simulink model "Copy_of_vehicle"  (R2021a)
settings: Solver=VariableStepAuto  StartTime=0  StopTime=80  RelTol=1e-3
values from neighbouring files (symbols this model uses):
  Ld = 0.3e-3    (= 0.0003)    [PMSM_paramaters.m]
  Lq = 0.4e-3    (= 0.0004)    [PMSM_paramaters.m]
  P = 4    [PMSM_paramaters.m]
  Pm = 0.15    [PMSM_paramaters.m]
  Rs = 0.03    [PMSM_paramaters.m]
  T_lookup = [289,289,0]    [PMSM_paramaters.m]
  Torque = 289    [PMSM_paramaters.m]
  Ts = 1e-2    (= 0.01)    [PMSM_paramaters.m]
undefined symbols (not defined in the file or in its folder): sigbuilder_block
libraries: pid_lib x3, simulink x3, autolibshared x1, simulink_extras x1, spspowerguiLib x1
settings Model: SimulationMode=accelerator  Creator=user  LastModifiedBy=USER
settings DebuggingCC: SFMachineParentedDataDiag=warning

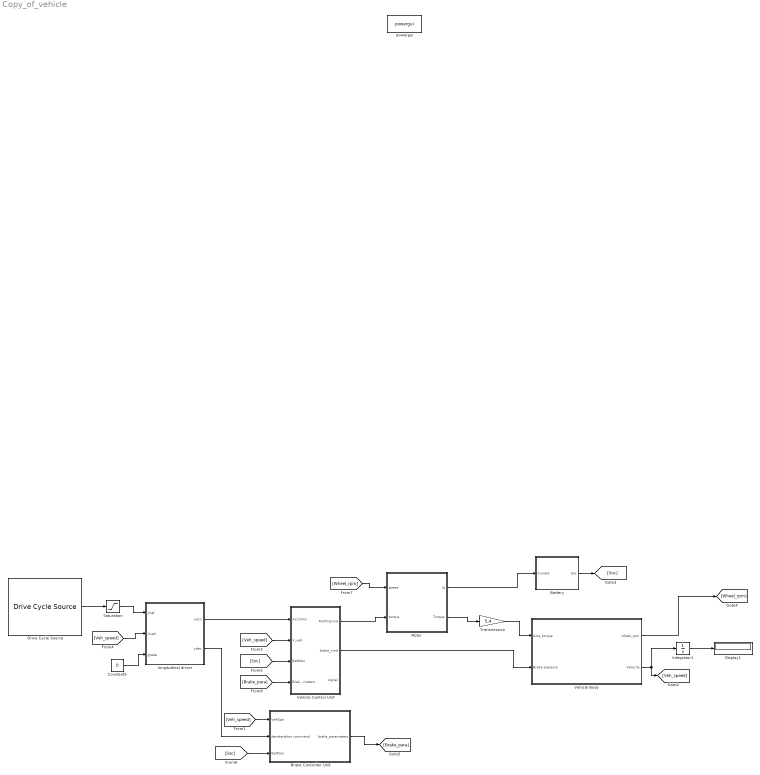
== system Copy_of_vehicle ==
  Battery : Subsystem
  Brake Controller Unit : Subsystem
  Constant5 : Constant  Value=0
  Display1 : Display
  Drive Cycle Source : autolibshared/Drive Cycle Source  cycleVar=Wide Open Throttle (WOT)  fileVar=cycleFTP75.mat  tfinal="300  seconds"  cycleRepeat=off  outAccPort=off  outGearPort=off  gearList=No gear data  t_wot1=0.1  xdot_woto=0  xdot_wot1=10.4  t_wot2=20  xdot_wot2=0  t_wotend=300  srcUnit=m/s  outUnit=m/s  srcAccUnit=m/s/s  outAccUnit=m/s^2  dt=0  aMode=1  faultOption=off  velBnd=2  velBndUnit=mph  inUnit=m/s  timeBnd=1  failOption=off  stopSim=off  maxFaultCnt=10  maxFaultTime=2  maxTotFaultTime=15  traceOption=off  dtTrace=1  traceWindow=10  lastDCname=Custom Data Set  lastOutUnit=mph  lastDT=0  lastTB=1  lastSB=2  forceCalcBound=off
      settings: SourceProductBaseCode=PW,DR,MT,UV,VE
  Integrator1 : Integrator
  Motor : Subsystem
  Saturation : Saturate  UpperLimit=50  LowerLimit=0
  Transmission : Gain  Gain=5.4
      settings: AttributesFormatString=%<Gain>
  Vehicle Body : Subsystem
  Vehicle Control Unit : Subsystem
  longitudinal driver : Subsystem
  powergui : spspowerguiLib/powergui  Priority=1  SimulationMode=Continuous  SampleTime=50e-6  frequency=60  Iterations=50  frequencyindice=0  Pbase=100e6  ErrMax=1e-4  UnitsV=kV  UnitsW=MW  buscounter=0  FunctionMessages=off  echomessages=off  EnableUseOfTLC=off  CurrentSourceSwitches=off  DisableSnubberDevices=off  DisableRonSwitches=off  DisableVfSwitches=off  DisplayEquations=off  AutomaticDiscreteSolvers=off  SolverType=Tustin/Backward Euler (TBE)  Interpol=off  ExternalGateDelay=off  methode=off  Ts=100  x0status=blocks  SPID=on  SwTol=0  HookPort=off  NonlinearTolerance=1e-4  nMaxIteration=100  ContinueOnMaxIteration=off  RestoreLinks=warning  ResistiveCurrentMeasurement=off  Frange=[0:2:500]  Ylog=off  Xlog=on  ShowGrid=off  save=off  variable=ZData  structure=0  ZoomFFT=off  StartTime=0.0  cycles=1  DisplayStyle=1  fundamental=60  FreqAxis=off  MaxFrequency=1000  frequencyindicesteady=1  RmsSteady=1  display=off
  wires:
  Drive Cycle Source/1 -> Saturation/1
  Integrator1/1 -> Display1/1
  Constant5/1 -> longitudinal driver/3(grade)
  Saturation/1 -> longitudinal driver/1(Vref)
  longitudinal driver/1(yacc) -> Vehicle Control Unit/1(AccCmd)
  longitudinal driver/2(ydec) -> Brake Controller Unit/2("deceleration command ")
  Vehicle Control Unit/2(brake_cmd) -> Vehicle Body/2(Brake pressure)
  Vehicle Body/2(Velocity) -> Integrator1/1, [Veh_speed]
  Transmission/1 -> Vehicle Body/1(Axle_torque)
  Vehicle Body/1(wheel_rpm) -> [Wheel_rpm]
  Brake Controller Unit/1(" brake_parameters") -> [Brake_para]
  Battery/1(Soc) -> [Soc]
  [Veh_speed] -> Brake Controller Unit/1(VehSpd)
  [Veh_speed] -> longitudinal driver/2(Vveh)
  [Veh_speed] -> Vehicle Control Unit/2(V_veh)
  [Soc] -> Vehicle Control Unit/3(BattSoc)
  [Soc] -> Brake Controller Unit/3(BattSoc)
  [Wheel_rpm] -> Motor/1(speed)
  Vehicle Control Unit/1(MotTrqCmd) -> Motor/2(torque)
  Motor/2(Torque) -> Transmission/1
  [Brake_para] -> Vehicle Control Unit/4(Brake_parameters)
  Motor/1(Iq) -> Battery/1(Current)

== system Copy_of_vehicle/Battery ==
  Current : Inport
  Constant : Constant
  Convert to Ah : Gain  Gain=-1/3600
  Convert to SOC : Gain  Gain=1/30200
  Integrator : Integrator
  e-ref : Sum
  Soc : Outport
  wires:
  Integrator/1 -> Convert to SOC/1
  Convert to Ah/1 -> Integrator/1
  Current/1 -> Convert to Ah/1
  Constant/1 -> e-ref/1
  Convert to SOC/1 -> e-ref/2
  e-ref/1 -> Soc/1

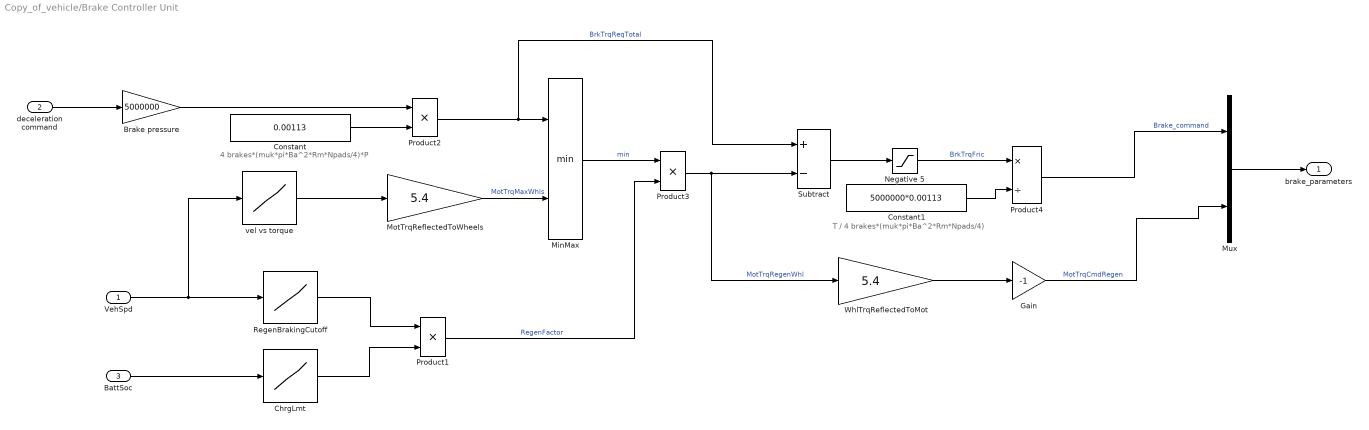
== system Copy_of_vehicle/Brake Controller Unit ==
  note: T / 4 brakes*(muk*pi*Ba^2*Rm*Npads/4)
  note: 4 brakes*(muk*pi*Ba^2*Rm*Npads/4)*P
  VehSpd : Inport
  "deceleration command " : Inport  Port=2
  BattSoc : Inport  Port=3
  Brake pressure : Gain  Gain=5000000
  ChrgLmt : Lookup_n-D  NumberOfTableDimensions=1  BreakpointsForDimension1=[0 10 20 30 40 50 60 70 80 90 100]  Table=[1 1 1 1 1 1 1 1 0.7 0.35 0]  ExtrapMethod=Clip  UseLastTableValue=on  InternalRulePriority=Speed  RndMeth=Simplest  InputSameDT=on
  Constant : Constant  Value=0.00113
  Constant1 : Constant  Value=5000000*0.00113
  Gain : Gain  Gain=-1
  MinMax : MinMax  Inputs=2
  MotTrqReflectedToWheels : Gain  Gain=5.4
  Mux : Mux  Inputs=2
  Negative 5 : Saturate  UpperLimit=inf  LowerLimit=0
  Product1 : Product
  Product2 : Product
  Product3 : Product
  Product4 : Product  Inputs=*/
  RegenBrakingCutoff : Lookup_n-D  NumberOfTableDimensions=1  BreakpointsForDimension1=[5 9]  Table=[0 1]  ExtrapMethod=Clip  UseLastTableValue=on  InternalRulePriority=Speed  RndMeth=Simplest  InputSameDT=on
  Subtract : Sum  Inputs=+-
  WhlTrqReflectedToMot : Gain  Gain=5.4
  vel vs torque : Lookup_n-D  NumberOfTableDimensions=1  BreakpointsForDimension1=[0 , 27.78,150]  Table=[286,286,0]  InternalRulePriority=Speed  RndMeth=Simplest  InputSameDT=on
  " brake_parameters" : Outport  VectorParamsAs1DForOutWhenUnconnected=off
  wires:
  Subtract/1 -> Negative 5/1
  Constant1/1 -> Product4/2
  MinMax/1 -> Product3/1  "min"
  BattSoc/1 -> ChrgLmt/1
  VehSpd/1 -> vel vs torque/1, RegenBrakingCutoff/1
  MotTrqReflectedToWheels/1 -> MinMax/2  "MotTrqMaxWhls"
  Constant/1 -> Product2/2
  "deceleration command "/1 -> Brake pressure/1
  Product2/1 -> MinMax/1, Subtract/1  "BrkTrqReqTotal"
  ChrgLmt/1 -> Product1/2
  RegenBrakingCutoff/1 -> Product1/1
  Product1/1 -> Product3/2  "RegenFactor"
  Negative 5/1 -> Product4/1  "BrkTrqFric"
  Mux/1 -> " brake_parameters"/1
  Product3/1 -> WhlTrqReflectedToMot/1, Subtract/2  "MotTrqRegenWhl"
  Gain/1 -> Mux/2  "MotTrqCmdRegen"
  WhlTrqReflectedToMot/1 -> Gain/1
  Product4/1 -> Mux/1  "Brake_command"
  Brake pressure/1 -> Product2/1
  vel vs torque/1 -> MotTrqReflectedToWheels/1

== system Copy_of_vehicle/Motor ==
  speed : Inport
  torque : Inport  Port=2
  1 : Gain  Gain=5.4
      settings: AttributesFormatString=%<Gain>
  FOC : Subsystem
  PMSM : Subsystem
  Unit Delay : UnitDelay  SampleTime=Ts  HasFrameUpgradeWarning=on
  Iq : Outport
  Torque : Outport  Port=2
  wires:
  torque/1 -> FOC/3(torque)
  FOC/1(Vabc) -> PMSM/1(Vabc)
  speed/1 -> 1/1
  PMSM/1(Iabc) -> FOC/2(Iabc)
  PMSM/3(Iq) -> Iq/1  "Iq"
  PMSM/2(Torque) -> Torque/1
  Unit Delay/1 -> FOC/4(Vdq)
  PMSM/4(Vdq) -> Unit Delay/1
  1/1 -> [Motor_speed]
  [Motor_speed] -> FOC/1(RotorSpeed_fbk)
  [Motor_speed] -> PMSM/2(speed)

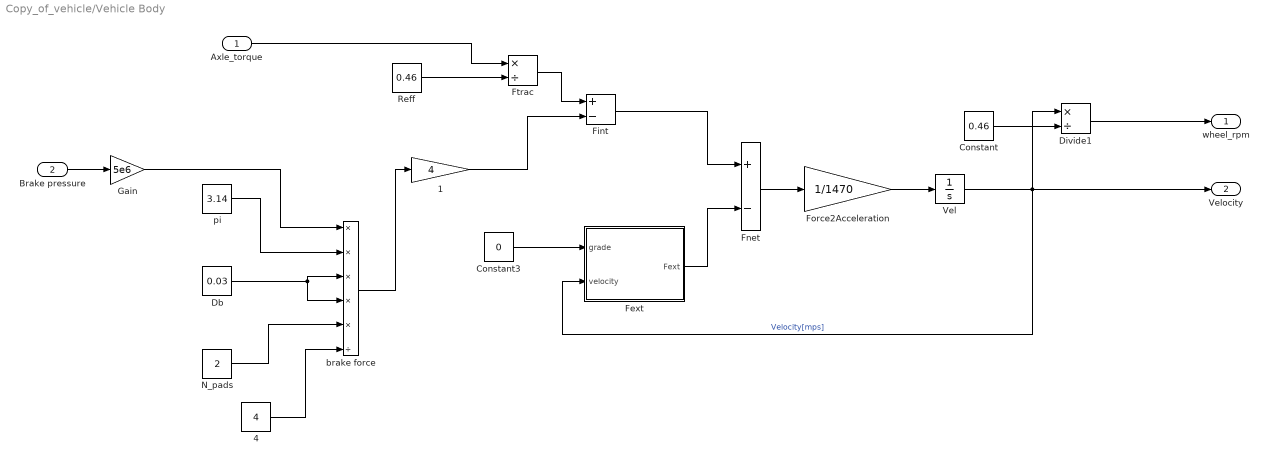
== system Copy_of_vehicle/Vehicle Body ==
  Axle_torque : Inport
  Brake pressure : Inport  Port=2
  1 : Gain  Gain=4
      settings: AttributesFormatString=%<Gain>
  4 : Constant  Value=4
  Constant : Constant  Value=0.46
  Constant3 : Constant  Value=0
  Db : Constant  Value=0.03
  Divide1 : Product  Inputs=*/
  Fext : Subsystem
  Fint : Sum  Inputs=+-
  Fnet : Sum  Inputs=+-
  Force2Acceleration : Gain  Gain=1/1470
      settings: AttributesFormatString=%<Gain>
  Ftrac : Product  Inputs=*/
  Gain : Gain  Gain=5e6
  N_pads : Constant  Value=2
  Reff : Constant  Value=0.46
  Vel : Integrator
  brake force : Product  Inputs=*****/
  pi : Constant  Value=3.14
  wheel_rpm : Outport
  Velocity : Outport  Port=2
  wires:
  Ftrac/1 -> Fint/1
  Fnet/1 -> Force2Acceleration/1
  Fext/1(Fext) -> Fnet/2
  Vel/1 -> Velocity/1, Divide1/1, Fext/2(velocity)  "Velocity[mps]"
  Reff/1 -> Ftrac/2
  Constant3/1 -> Fext/1(grade)
  Brake pressure/1 -> Gain/1
  Fint/1 -> Fnet/1
  Axle_torque/1 -> Ftrac/1
  1/1 -> Fint/2
  Force2Acceleration/1 -> Vel/1
  Constant/1 -> Divide1/2
  Divide1/1 -> wheel_rpm/1
  brake force/1 -> 1/1
  Gain/1 -> brake force/1
  4/1 -> brake force/6
  Db/1 -> brake force/3, brake force/4
  pi/1 -> brake force/2
  N_pads/1 -> brake force/5

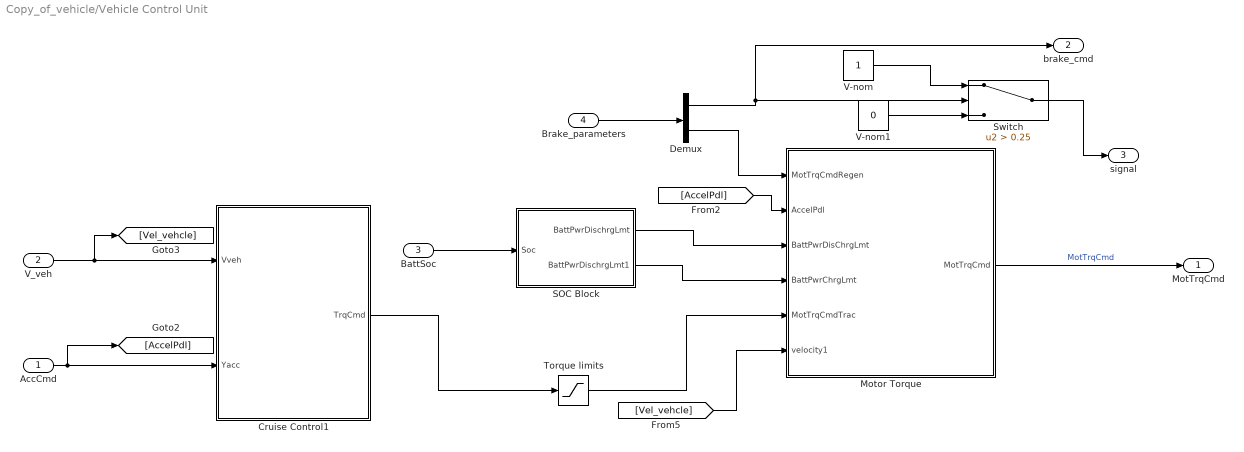
== system Copy_of_vehicle/Vehicle Control Unit ==
  AccCmd : Inport
  V_veh : Inport  Port=2
  BattSoc : Inport  Port=3
  Brake_parameters : Inport  Port=4
  Cruise Control1 : Subsystem
  Demux : Demux  Outputs=2
  "Motor Torque " : Subsystem
  SOC Block : Subsystem
  Switch : Switch  Criteria=u2 > Threshold  Threshold=0.25
  Torque limits : Saturate  UpperLimit=Torque  LowerLimit=0
  V-nom : Constant
  V-nom1 : Constant  Value=0
  MotTrqCmd : Outport
  brake_cmd : Outport  Port=2
  signal : Outport  Port=3
  wires:
  Torque limits/1 -> "Motor Torque "/5(MotTrqCmdTrac)
  V_veh/1 -> Cruise Control1/1(Vveh), [Vel_vehcle]
  Cruise Control1/1(TrqCmd) -> Torque limits/1
  AccCmd/1 -> Cruise Control1/2(Yacc), [AccelPdl]
  SOC Block/1(BattPwrDischrgLmt) -> "Motor Torque "/3(BattPwrDisChrgLmt)
  BattSoc/1 -> SOC Block/1(Soc)
  SOC Block/2(BattPwrDischrgLmt1) -> "Motor Torque "/4("BattPwrChrgLmt ")
  "Motor Torque "/1(MotTrqCmd) -> MotTrqCmd/1  "MotTrqCmd"
  [Vel_vehcle] -> "Motor Torque "/6(velocity1)
  [AccelPdl] -> "Motor Torque "/2(AccelPdl)
  Brake_parameters/1 -> Demux/1
  Demux/2 -> "Motor Torque "/1(MotTrqCmdRegen)
  Demux/1 -> brake_cmd/1, Switch/2
  V-nom1/1 -> Switch/3
  V-nom/1 -> Switch/1
  Switch/1 -> signal/1

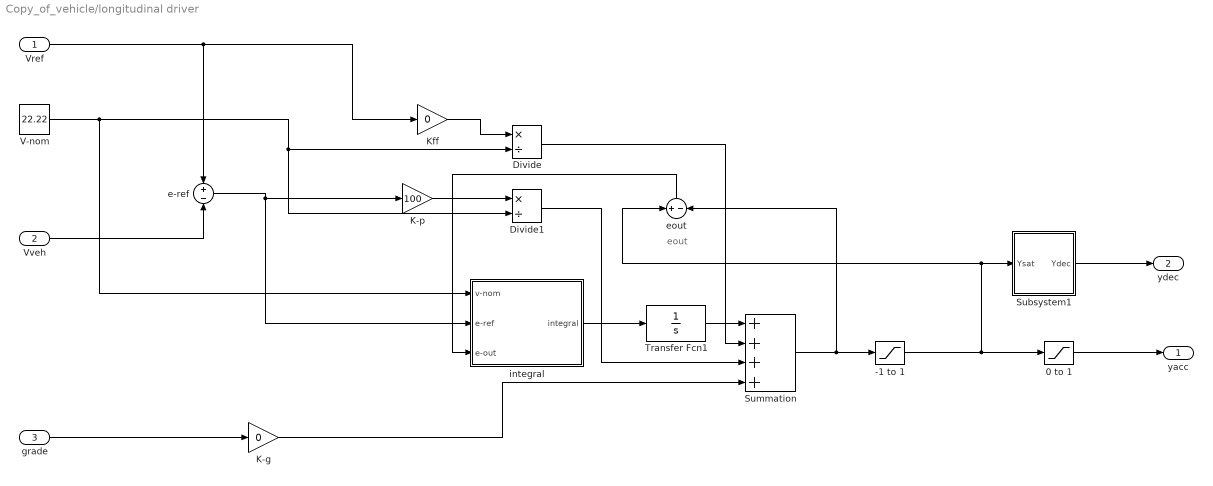
== system Copy_of_vehicle/longitudinal driver ==
  note: eout
  Vref : Inport
  Vveh : Inport  Port=2
  grade : Inport  Port=3
  "-1 to 1 " : Saturate  UpperLimit=1  LowerLimit=-1
  0 to 1 : Saturate  UpperLimit=1  LowerLimit=0
  Divide : Product  Inputs=*/
  Divide1 : Product  Inputs=*/
  K-g : Gain  Gain=0
  K-p : Gain  Gain=100
  Kff : Gain  Gain=0
  Subsystem1 : Subsystem
  Summation : Sum  Inputs=++++
  Transfer Fcn1 : TransferFcn  Denominator=[1 0]
  V-nom : Constant  Value=22.22
  e-ref : Sum  Inputs=+-
  eout : Sum  Inputs=+-
  integral : Subsystem
  yacc : Outport
  ydec : Outport  Port=2
  wires:
  V-nom/1 -> Divide1/2, Divide/2, integral/1(v-nom)
  e-ref/1 -> K-p/1, integral/2(e-ref)
  Divide/1 -> Summation/2
  Summation/1 -> "-1 to 1 "/1, eout/2
  Vref/1 -> Kff/1, e-ref/1
  integral/1(integral) -> Transfer Fcn1/1
  K-p/1 -> Divide1/1
  Transfer Fcn1/1 -> Summation/1
  Kff/1 -> Divide/1
  eout/1 -> integral/3(e-out)
  Vveh/1 -> e-ref/2
  Divide1/1 -> Summation/3
  grade/1 -> K-g/1
  Subsystem1/1(Ydec) -> ydec/1
  0 to 1/1 -> yacc/1
  K-g/1 -> Summation/4
  "-1 to 1 "/1 -> 0 to 1/1, Subsystem1/1(Ysat), eout/1

== system Copy_of_vehicle/Motor/FOC ==
  RotorSpeed_fbk : Inport
  Iabc : Inport  Port=2
  torque : Inport  Port=3
  Vdq : Inport  Port=4
  Inverse - Park1 : Subsystem
  Inverse Clarke1 : Subsystem
  Subsystem2 : Subsystem
  clarke : Subsystem
  current controller : Subsystem
  park : Subsystem
  torque_Idq_ref : Subsystem
  Vabc : Outport
  wires:
  [theta] -> Inverse - Park1/2(theta)
  RotorSpeed_fbk/1 -> [Omega], Subsystem2/1(omega)
  Inverse - Park1/2(V-beta) -> Inverse Clarke1/2(Vbeta)
  Iabc/1 -> clarke/1(Iabc)
  torque/1 -> torque_Idq_ref/1(Torque)
  Inverse - Park1/1(V-alpha) -> Inverse Clarke1/1(Valpha)
  current controller/2(Vq) -> Inverse - Park1/3(Vq)
  park/1(Id) -> current controller/2(Id), torque_Idq_ref/2(Id)
  current controller/1(Vd) -> Inverse - Park1/1(Vd)
  Subsystem2/1(theta_deg) -> park/2(theta), [theta]
  torque_Idq_ref/1(Id_ref) -> current controller/1(Id_ref)
  park/2(Iq) -> current controller/4(Iq)
  [Omega] -> current controller/3(omega)
  torque_Idq_ref/2(Iq_ref) -> current controller/5(Iq_ref)
  clarke/1(I_alpha) -> park/1(I_alpha)
  Inverse Clarke1/1(Vabc) -> Vabc/1
  clarke/2(I_beta) -> park/3(I_beta)
  Vdq/1 -> torque_Idq_ref/3(Vdq)

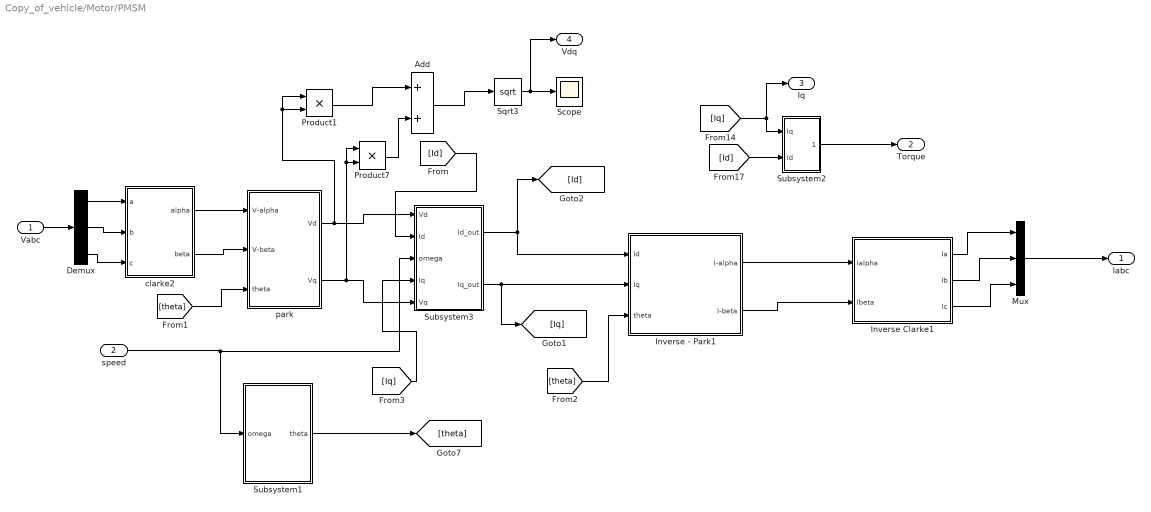
== system Copy_of_vehicle/Motor/PMSM ==
  Vabc : Inport
  speed : Inport  Port=2
  Add : Sum
  Demux : Demux  Outputs=3
  Inverse - Park1 : Subsystem
  Inverse Clarke1 : Subsystem
  Mux : Mux  Inputs=3
  Product1 : Product
  Product7 : Product
  Scope : Scope
  Sqrt3 : Sqrt  SaturateOnIntegerOverflow=on
  Subsystem1 : Subsystem
  Subsystem2 : Subsystem
  Subsystem3 : Subsystem
  clarke2 : Subsystem
  park : Subsystem
  Iabc : Outport
  Torque : Outport  Port=2
  Iq : Outport  Port=3
  Vdq : Outport  Port=4
  wires:
  Mux/1 -> Iabc/1
  Demux/1 -> clarke2/1(a)
  Vabc/1 -> Demux/1
  Inverse - Park1/2(I-beta) -> Inverse Clarke1/2(Ibeta)
  Subsystem3/1(Id_out) -> Inverse - Park1/1(Id), [Id]
  Inverse Clarke1/1(Ia) -> Mux/1
  Demux/3 -> clarke2/3(c)
  Demux/2 -> clarke2/2(b)
  Subsystem1/1(theta) -> [theta]
  Inverse Clarke1/2(Ib) -> Mux/2
  clarke2/2(beta) -> park/2(V-beta)
  [Id] -> Subsystem3/2(Id)
  Subsystem3/2(Iq_out) -> Inverse - Park1/2(Iq), [Iq]
  clarke2/1(alpha) -> park/1(V-alpha)
  park/2(Vq) -> Subsystem3/5(Vq), Product7/1, Product7/2
  Inverse Clarke1/3(Ic) -> Mux/3
  Inverse - Park1/1(I-alpha) -> Inverse Clarke1/1(Ialpha)
  park/1(Vd) -> Product1/2, Product1/1, Subsystem3/1(Vd)
  [Id] -> Subsystem2/2(Id)
  [theta] -> park/3(theta)
  [Iq] -> Iq/1, Subsystem2/1(Iq)
  Subsystem2/1(Torque) -> Torque/1
  [theta] -> Inverse - Park1/3(theta)
  speed/1 -> Subsystem1/1(omega), Subsystem3/3(omega)
  [Iq] -> Subsystem3/4(Iq)
  Product7/1 -> Add/2
  Product1/1 -> Add/1
  Add/1 -> Sqrt3/1
  Sqrt3/1 -> Vdq/1, Scope/1

== system Copy_of_vehicle/Vehicle Body/Fext ==
  grade : Inport
  velocity : Inport  Port=2
  Cd1 : Constant  Value=0.38  OutDataTypeStr=single
  Cd2 : Constant  Value=2.27  OutDataTypeStr=single
  Cos : Trigonometry  Operator=cos
  Sum : Sum  Inputs=+++
  Trigonometric Function : Trigonometry
  aero : Product  Inputs=6
  coeff_fric : Constant  Value=0.01  OutDataTypeStr=single
  constant : Constant  Value=0.5  OutDataTypeStr=single
  density : Constant  Value=1.2  OutDataTypeStr=single
  g : Constant  Value=9.81  OutDataTypeStr=single
  g1 : Constant  OutDataTypeStr=single
  g2 : Constant  Value=9.81  OutDataTypeStr=single
  gradient_force : Product  Inputs=3
  mass : Constant  Value=1470  OutDataTypeStr=single
  rolling_res : Product  Inputs=5
  Fext : Outport
  wires:
  g2/1 -> gradient_force/2
  mass/1 -> gradient_force/3, rolling_res/1
  Trigonometric Function/1 -> gradient_force/1
  g/1 -> rolling_res/2
  g1/1 -> rolling_res/3
  grade/1 -> Cos/1, Trigonometric Function/1
  coeff_fric/1 -> rolling_res/4
  Cd1/1 -> aero/4
  density/1 -> aero/2
  constant/1 -> aero/1
  Cd2/1 -> aero/5
  velocity/1 -> aero/3, aero/6
  gradient_force/1 -> Sum/1
  aero/1 -> Sum/2
  rolling_res/1 -> Sum/3
  Sum/1 -> Fext/1
  Cos/1 -> rolling_res/5

== system Copy_of_vehicle/Vehicle Control Unit/Cruise Control1 ==
  Vveh : Inport
  Yacc : Inport  Port=2
  Capture speed : Subsystem  TreatAsAtomicUnit=on
  Constant5 : Constant  Value=0
  Data Type Conversion1 : DataTypeConversion  OutDataTypeStr=boolean
  Data Type Conversion2 : DataTypeConversion  OutDataTypeStr=boolean
  Data Type Conversion3 : DataTypeConversion  OutDataTypeStr=boolean
  Inputs1 : Subsystem  Tag=STV Subsys  LoadFcn=sigbuilder_block('load');  StartFcn=sigbuilder_block('start');  StopFcn=sigbuilder_block('stop');  ClipboardFcn=sigbuilder_block('clipboard');  mask(Sigbuilder block){tuvar=[0:10]}
      mask help: Simulink:masks:SigbuilderBlock_MD
      mask init:
      | if ~strcmp(get_param(bdroot(gcbh),'SimulationStatus'),'stopped') tuvar = sigbuilder_block('maskInit'); end
      settings: CopyFcn=sigbuilder_block('copy');  DeleteFcn=sigbuilder_block('delete');  ModelCloseFcn=sigbuilder_block('modelClose');  PreSaveFcn=sigbuilder_block('preSave');  PauseFcn=sigbuilder_block('pause');  ContinueFcn=sigbuilder_block('continue');  NameChangeFcn=sigbuilder_block('namechange');  OpenFcn=sigbuilder_block('open',[5.4 30 1141.2 522.6 ]);  CloseFcn=sigbuilder_block('close');
      mask Display: plot(0, 0, 100, 100,[2, 2, 32, 32, 2], [68, 8, 8, 68, 68],[32, 2], [38, 38], [32, 19, 2],[53, 60, 44], [32, 17, 17, 2],[16, 16, 31, 31]);txt = getActiveGroup(gcbh);text(2, 100, txt,'verticalAlignment', 'top');
  J-K Flip-Flop : simulink_extras/Flip Flops/J-K Flip-Flop  initial_condition=0
      settings: SourceProductName=Simulink Extras
  Pulse Generator : DiscretePulseGenerator  Period=10  PulseWidth=5  SampleTime=0.01
  Subsystem : Subsystem
  Switch : Switch  Criteria=u2 > Threshold
  Terminator : Terminator
  longitudinal driver : Subsystem
  TrqCmd : Outport  VectorParamsAs1DForOutWhenUnconnected=off
  wires:
  Inputs1/1(Cruise Ena.) -> Data Type Conversion1/1
  Pulse Generator/1 -> Data Type Conversion2/1
  J-K Flip-Flop/1 -> Switch/2, Capture speed/Trigger
  Data Type Conversion1/1 -> J-K Flip-Flop/1
  J-K Flip-Flop/2 -> Terminator/1
  Capture speed/1(Vref) -> longitudinal driver/1(Vref)
  Inputs1/2(Cruise Dis.) -> Data Type Conversion3/1
  Yacc/1 -> Switch/3
  longitudinal driver/1(yacc) -> Switch/1
  Constant5/1 -> longitudinal driver/3(grade)
  Switch/1 -> Subsystem/1(Acc_pedal)
  Vveh/1 -> Capture speed/1(Vveh), Subsystem/2(velocity), longitudinal driver/2(Vveh)
  Subsystem/1(Torque_cmd) -> TrqCmd/1
  Data Type Conversion2/1 -> J-K Flip-Flop/2
  Data Type Conversion3/1 -> J-K Flip-Flop/3

== system Copy_of_vehicle/Vehicle Control Unit/Motor Torque  ==
  MotTrqCmdRegen : Inport
  AccelPdl : Inport  Port=2
  BattPwrDisChrgLmt : Inport  Port=3
  "BattPwrChrgLmt " : Inport  Port=4
  MotTrqCmdTrac : Inport  Port=5
  velocity1 : Inport  Port=6
  Accel Decel Switch : Switch  Criteria=u2 > Threshold
  Compare To Constant : simulink/Logic and Bit Operations/Compare To Constant  relop=>  const=0  OutDataTypeStr=boolean
  Gain : Gain  Gain=-1
  Saturation Dynamic : simulink/Discontinuities/Saturation Dynamic  OutMin=[]  OutMax=[]  OutDataTypeStr=Inherit: Same as second input  OutDataType=fixdt(1, 16)  OutScaling=2^-10  DoSatur=off
  Saturation Dynamic1 : simulink/Discontinuities/Saturation Dynamic  OutMin=[]  OutMax=[]  OutDataTypeStr=Inherit: Same as second input  OutDataType=fixdt(1, 16)  OutScaling=2^-10  DoSatur=off
  Vel vs Torque : Lookup_n-D  NumberOfTableDimensions=1  BreakpointsForDimension1=[0 , 27.78,50]  Table=T_lookup  InternalRulePriority=Speed  RndMeth=Simplest  InputSameDT=on
  MotTrqCmd : Outport
  wires:
  AccelPdl/1 -> Compare To Constant/1
  MotTrqCmdRegen/1 -> Accel Decel Switch/3
  MotTrqCmdTrac/1 -> Accel Decel Switch/1
  Accel Decel Switch/1 -> Saturation Dynamic1/2
  Compare To Constant/1 -> Accel Decel Switch/2
  Gain/1 -> Saturation Dynamic/3
  "BattPwrChrgLmt "/1 -> Saturation Dynamic1/3
  BattPwrDisChrgLmt/1 -> Saturation Dynamic1/1
  Saturation Dynamic1/1 -> Saturation Dynamic/2
  velocity1/1 -> Vel vs Torque/1
  Saturation Dynamic/1 -> MotTrqCmd/1
  Vel vs Torque/1 -> Saturation Dynamic/1, Gain/1

== system Copy_of_vehicle/Vehicle Control Unit/SOC Block ==
  Soc : Inport
  ChrgLmt : Lookup_n-D  NumberOfTableDimensions=1  BreakpointsForDimension1=[0 10 20 30 40 50 60 70 80 90 100]  Table=[1 1 1 1 1 1 1 1 0.7 0.35 0]  ExtrapMethod=Clip  UseLastTableValue=on  InternalRulePriority=Speed  RndMeth=Simplest  InputSameDT=on
  DischrgLmt : Lookup_n-D  NumberOfTableDimensions=1  BreakpointsForDimension1=[0 10 20 30 40 50 60 70 80 90 100]  Table=[0 0.35 0.7 1 1 1 1 1 1 1 1]  ExtrapMethod=Clip  UseLastTableValue=on  InternalRulePriority=Speed  RndMeth=Simplest  InputSameDT=on
  MaxChrg : Constant  Value=96234
  MaxChrg1 : Constant  Value=-96234
  Product : Product
  Product1 : Product
  BattPwrDischrgLmt : Outport  VectorParamsAs1DForOutWhenUnconnected=off
  BattPwrDischrgLmt1 : Outport  Port=2  VectorParamsAs1DForOutWhenUnconnected=off
  wires:
  Soc/1 -> DischrgLmt/1, ChrgLmt/1
  Product1/1 -> BattPwrDischrgLmt1/1
  Product/1 -> BattPwrDischrgLmt/1
  MaxChrg1/1 -> Product1/2
  ChrgLmt/1 -> Product1/1
  MaxChrg/1 -> Product/2
  DischrgLmt/1 -> Product/1

== system Copy_of_vehicle/longitudinal driver/Subsystem1 ==
  Ysat : Inport
  -2 : Constant  Value=0
  -5 : Constant
  K-p1 : Gain  Gain=-1
  K-p2 : Gain  Gain=-1
  Switch5 : Switch  Criteria=u2 > Threshold
  Switch6 : Switch  Threshold=-1
  Ydec : Outport
  wires:
  Switch5/1 -> Switch6/1, K-p2/1
  K-p1/1 -> Switch5/3
  Switch6/1 -> Ydec/1
  Ysat/1 -> Switch5/2, K-p1/1
  K-p2/1 -> Switch6/2
  -2/1 -> Switch5/1
  -5/1 -> Switch6/3

== system Copy_of_vehicle/longitudinal driver/integral ==
  v-nom : Inport
  e-ref : Inport  Port=2
  e-out : Inport  Port=3
  Divide2 : Product  Inputs=*/
  K-aw : Gain  Gain=0
  Ki : Gain
  Sum2 : Sum  Inputs=|++
  integral : Outport
  wires:
  Divide2/1 -> Sum2/1
  v-nom/1 -> Divide2/2
  e-ref/1 -> Ki/1
  K-aw/1 -> Sum2/2
  Ki/1 -> Divide2/1
  e-out/1 -> K-aw/1
  Sum2/1 -> integral/1

== system Copy_of_vehicle/Motor/FOC/Inverse - Park1 ==
  Vd : Inport
  theta : Inport  Port=2
  Vq : Inport  Port=3
  Cos : Trigonometry  Operator=cos
  Product{,1..3} (4 alike) : Product
  Sin : Trigonometry
  Sum3 : Sum  Inputs=|++
  Sum4 : Sum  Inputs=+-
  V-alpha : Outport
  V-beta : Outport  Port=2
  wires:
  Vq/1 -> Product2/1, Product1/1
  Cos/1 -> Product1/2, Product3/2
  Sin/1 -> Product/2, Product2/2
  Product/1 -> Sum3/2
  Product3/1 -> Sum4/1
  Sum3/1 -> V-beta/1
  Product1/1 -> Sum3/1
  Product2/1 -> Sum4/2
  Vd/1 -> Product3/1, Product/1
  Sum4/1 -> V-alpha/1
  theta/1 -> Cos/1, Sin/1

== system Copy_of_vehicle/Motor/FOC/Inverse Clarke1 ==
  Valpha : Inport
  Vbeta : Inport  Port=2
  Constant : Constant  Value=0.5  OutDataTypeStr=single
  Constant18 : Constant  Value=3/4  OutDataTypeStr=single
  Mux : Mux  Inputs=3
  Product8 : Product
  Product9 : Product
  Sqrt : Sqrt  SaturateOnIntegerOverflow=on
  Sum : Sum  Inputs=-+
  Sum1 : Sum  Inputs=--
  Sum7 : Sum  Inputs=|++
  Vabc : Outport
  wires:
  Product9/1 -> Sum1/2, Sum/2
  Product8/1 -> Sum7/1, Sum1/1, Sum7/2, Sum/1
  Constant18/1 -> Sqrt/1
  Sum/1 -> Mux/2
  Vbeta/1 -> Product9/1
  Sum7/1 -> Mux/1
  Constant/1 -> Product8/2
  Sqrt/1 -> Product9/2
  Sum1/1 -> Mux/3
  Valpha/1 -> Product8/1
  Mux/1 -> Vabc/1

== system Copy_of_vehicle/Motor/FOC/Subsystem2 ==
  omega : Inport
  Constant8 : Constant  Value=2*pi
  Gain4 : Gain  Gain=0.5
  Integrator2 : Integrator
  Math Function : Math  Operator=mod  SaturateOnIntegerOverflow=on
  P : Constant  Value=P
  Product15 : Product
  Unit Delay : UnitDelay  SampleTime=Ts  HasFrameUpgradeWarning=on
  theta_deg : Outport
  wires:
  omega/1 -> Product15/1
  P/1 -> Gain4/1
  Product15/1 -> Unit Delay/1
  Gain4/1 -> Product15/2
  Unit Delay/1 -> Integrator2/1
  Constant8/1 -> Math Function/2
  Integrator2/1 -> Math Function/1
  Math Function/1 -> theta_deg/1

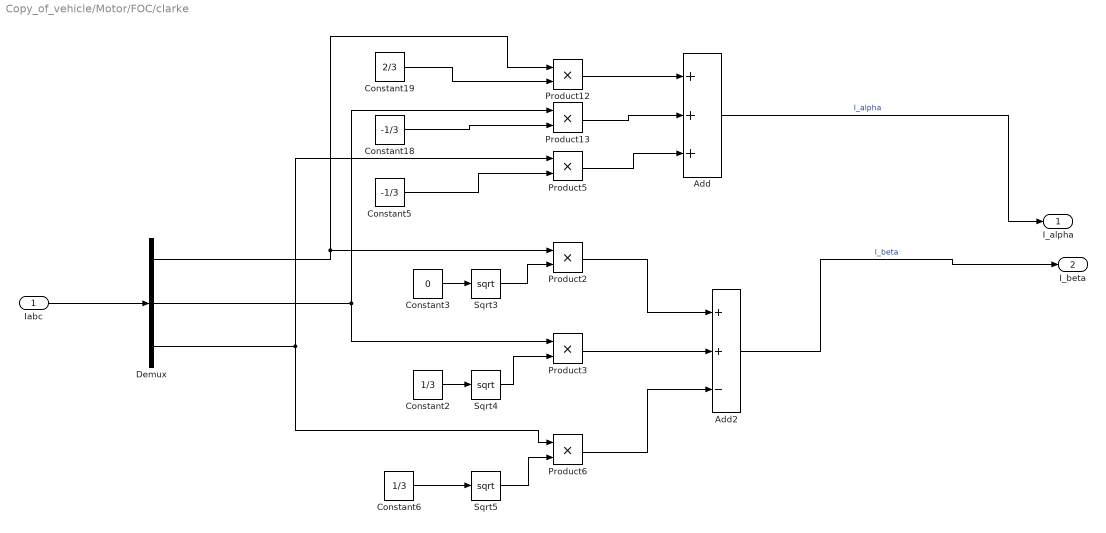
== system Copy_of_vehicle/Motor/FOC/clarke ==
  Iabc : Inport
  Add : Sum  Inputs=+++
  Add2 : Sum  Inputs=++-
  Constant18 : Constant  Value=-1/3  OutDataTypeStr=single
  Constant19 : Constant  Value=2/3  OutDataTypeStr=single
  Constant2 : Constant  Value=1/3  OutDataTypeStr=single
  Constant3 : Constant  Value=0  OutDataTypeStr=single
  Constant5 : Constant  Value=-1/3  OutDataTypeStr=single
  Constant6 : Constant  Value=1/3  OutDataTypeStr=single
  Demux : Demux  Outputs=3
  Product{2..3,5..6,12..13} (6 alike) : Product
  Sqrt3 : Sqrt  SaturateOnIntegerOverflow=on
  Sqrt4 : Sqrt  SaturateOnIntegerOverflow=on
  Sqrt5 : Sqrt  SaturateOnIntegerOverflow=on
  I_alpha : Outport
  I_beta : Outport  Port=2
  wires:
  Constant19/1 -> Product12/2
  Constant18/1 -> Product13/2
  Constant3/1 -> Sqrt3/1
  Sqrt4/1 -> Product3/2
  Constant2/1 -> Sqrt4/1
  Sqrt3/1 -> Product2/2
  Demux/1 -> Product12/1, Product2/1
  Demux/2 -> Product3/1, Product13/1
  Constant5/1 -> Product5/2
  Demux/3 -> Product6/1, Product5/1
  Constant6/1 -> Sqrt5/1
  Sqrt5/1 -> Product6/2
  Product12/1 -> Add/1
  Product13/1 -> Add/2
  Product2/1 -> Add2/1
  Product3/1 -> Add2/2
  Product6/1 -> Add2/3
  Add/1 -> I_alpha/1  "I_alpha"
  Add2/1 -> I_beta/1  "I_beta"
  Product5/1 -> Add/3
  Iabc/1 -> Demux/1

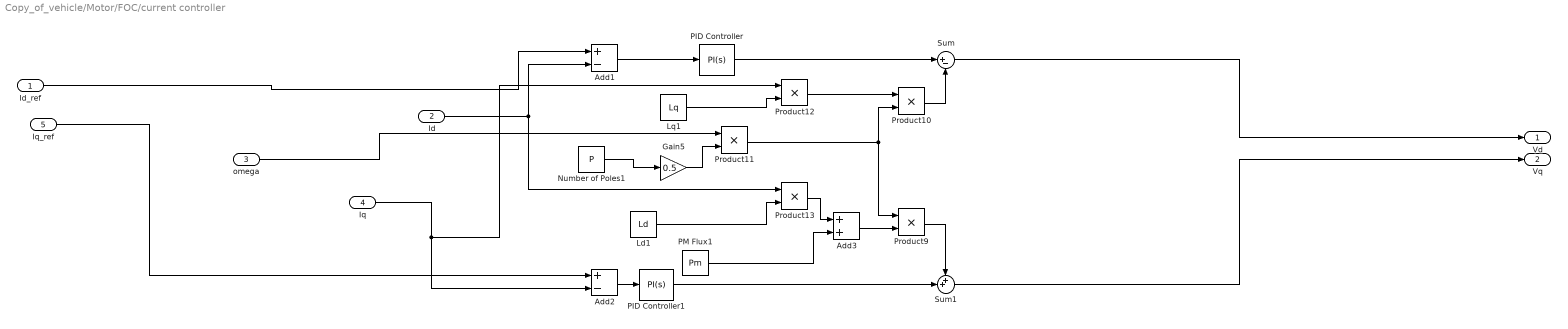
== system Copy_of_vehicle/Motor/FOC/current controller ==
  Id_ref : Inport
  Id : Inport  Port=2
  omega : Inport  Port=3
  Iq : Inport  Port=4
  Iq_ref : Inport  Port=5
  Add1 : Sum  Inputs=+-  OutDataTypeStr=double
  Add2 : Sum  Inputs=+-
  Add3 : Sum
  Gain5 : Gain  Gain=0.5
  Ld1 : Constant  Value=Ld
  Lq1 : Constant  Value=Lq
  Number of Poles1 : Constant  Value=P
  PID Controller : pid_lib/PID Controller  Controller=PI  Form=Ideal  TimeDomain=Continuous-time  UseExternalTs=off  SampleTime=Ts  IntegratorMethod=Forward Euler  FilterMethod=Forward Euler  ControllerParametersSource=internal  P=200  I=1  D=0  UseFilter=on  N=100  TunerSelectOption=Transfer Function Based (PID Tuner App)  InitialConditionSource=internal  InitialConditionForIntegrator=0  InitialConditionForFilter=0  DifferentiatorICPrevScaledInput=0  ExternalReset=none  TrackingMode=off  Kt=1  LimitOutput=on  SatLimitsSource=internal  UpperSaturationLimit=320  LowerSaturationLimit=-320  LinearizeAsGain=on  AntiWindupMode=none  Kb=1  POutMin=[]  POutMax=[]  IOutMin=[]  IOutMax=[]  DOutMin=[]  DOutMax=[]  NOutMin=[]  NOutMax=[]  SumOutMin=[]  SumOutMax=[]  SaturationOutMin=[]  SaturationOutMax=[]  PParamMin=[]  PParamMax=[]  IParamMin=[]  IParamMax=[]  DParamMin=[]  DParamMax=[]  NParamMin=[]  NParamMax=[]  KbParamMin=[]  KbParamMax=[]  KtParamMin=[]  KtParamMax=[]  KbOutMin=[]  KbOutMax=[]  KtOutMin=[]  KtOutMax=[]  IntegratorOutMin=[]  IntegratorOutMax=[]  FilterOutMin=[]  FilterOutMax=[]  SumI1OutMin=[]  SumI1OutMax=[]  SumI2OutMin=[]  SumI2OutMax=[]  SumI3OutMin=[]  SumI3OutMax=[]  SumI4OutMin=[]  SumI4OutMax=[]  SumDOutMin=[]  SumDOutMax=[]  DifferentiatorOutMin=[]  DifferentiatorOutMax=[]  FilterDiffOutCoefMin=[]  FilterDiffOutCoefMax=[]  ReciprocalOutMin=[]  ReciprocalOutMax=[]  SumDenOutMin=[]  SumDenOutMax=[]  SumNumOutMin=[]  SumNumOutMax=[]  DivideOutMin=[]  DivideOutMax=[]  UdiffTsProdOutMin=[]  UdiffTsProdOutMax=[]  NTsProdOutMin=[]  NTsProdOutMax=[]  UintegralTsProdOutMin=[]  UintegralTsProdOutMax=[]  UngainTsProdOutMin=[]  UngainTsProdOutMax=[]  IntegratorContinuousStateAttributes=''  IntegratorStateMustResolveToSignalObject=off  IntegratorRTWStateStorageClass=Auto  FilterContinuousStateAttributes=''  FilterStateMustResolveToSignalObject=off  FilterRTWStateStorageClass=Auto  ParallelPVariant=Passthrough  IdealPVariant=InternalParameters  IVariant=InternalParameters  DVariant=Disabled  IntegratorVariant=Continuous  SatVariant=Enabled  AWVariant=Passthrough  PCopyVariant=Disabled  TRVariant=Disabled  FdbkBlocksVariant=Forward  IdealPFdbkVariant=Disabled  SatFdbkVariant=Disabled  DerivativeFilterVariant=Disabled  NVariant=Disabled  NCopyVariant=Disabled_SignalSpec  FilterICVariant=Disabled  IntegratorICVariant=InternalICs  ExternalResetVariant=Disabled  TRSumVariant=Passthrough  SumFdbkVariant=Disabled  SumVariant=Sum_PI  TsampFilterVariant=InternalTs  TsampNgainVariant=Passthrough  TsampIntegralVariant=Passthrough  ExternalSaturationOutDataTypeStr=Inherit: Same as second input
  PID Controller1 : pid_lib/PID Controller  Controller=PI  Form=Parallel  TimeDomain=Continuous-time  UseExternalTs=off  SampleTime=Ts  IntegratorMethod=Forward Euler  FilterMethod=Forward Euler  ControllerParametersSource=internal  P=200  I=1  D=0  UseFilter=on  N=100  TunerSelectOption=Transfer Function Based (PID Tuner App)  InitialConditionSource=internal  InitialConditionForIntegrator=0  InitialConditionForFilter=0  DifferentiatorICPrevScaledInput=0  ExternalReset=none  TrackingMode=off  Kt=1  LimitOutput=on  SatLimitsSource=internal  UpperSaturationLimit=320  LowerSaturationLimit=-320  LinearizeAsGain=on  AntiWindupMode=none  Kb=1  POutMin=[]  POutMax=[]  IOutMin=[]  IOutMax=[]  DOutMin=[]  DOutMax=[]  NOutMin=[]  NOutMax=[]  SumOutMin=[]  SumOutMax=[]  SaturationOutMin=[]  SaturationOutMax=[]  PParamMin=[]  PParamMax=[]  IParamMin=[]  IParamMax=[]  DParamMin=[]  DParamMax=[]  NParamMin=[]  NParamMax=[]  KbParamMin=[]  KbParamMax=[]  KtParamMin=[]  KtParamMax=[]  KbOutMin=[]  KbOutMax=[]  KtOutMin=[]  KtOutMax=[]  IntegratorOutMin=[]  IntegratorOutMax=[]  FilterOutMin=[]  FilterOutMax=[]  SumI1OutMin=[]  SumI1OutMax=[]  SumI2OutMin=[]  SumI2OutMax=[]  SumI3OutMin=[]  SumI3OutMax=[]  SumI4OutMin=[]  SumI4OutMax=[]  SumDOutMin=[]  SumDOutMax=[]  DifferentiatorOutMin=[]  DifferentiatorOutMax=[]  FilterDiffOutCoefMin=[]  FilterDiffOutCoefMax=[]  ReciprocalOutMin=[]  ReciprocalOutMax=[]  SumDenOutMin=[]  SumDenOutMax=[]  SumNumOutMin=[]  SumNumOutMax=[]  DivideOutMin=[]  DivideOutMax=[]  UdiffTsProdOutMin=[]  UdiffTsProdOutMax=[]  NTsProdOutMin=[]  NTsProdOutMax=[]  UintegralTsProdOutMin=[]  UintegralTsProdOutMax=[]  UngainTsProdOutMin=[]  UngainTsProdOutMax=[]  IntegratorContinuousStateAttributes=''  IntegratorStateMustResolveToSignalObject=off  IntegratorRTWStateStorageClass=Auto  FilterContinuousStateAttributes=''  FilterStateMustResolveToSignalObject=off  FilterRTWStateStorageClass=Auto  ParallelPVariant=InternalParameters  IdealPVariant=Disabled  IVariant=InternalParameters  DVariant=Disabled  IntegratorVariant=Continuous  SatVariant=Enabled  AWVariant=Passthrough  PCopyVariant=Disabled  TRVariant=Disabled  FdbkBlocksVariant=Forward  IdealPFdbkVariant=Disabled  SatFdbkVariant=Disabled  DerivativeFilterVariant=Disabled  NVariant=Disabled  NCopyVariant=Disabled_SignalSpec  FilterICVariant=Disabled  IntegratorICVariant=InternalICs  ExternalResetVariant=Disabled  TRSumVariant=Passthrough  SumFdbkVariant=Disabled  SumVariant=Sum_PI  TsampFilterVariant=InternalTs  TsampNgainVariant=Passthrough  TsampIntegralVariant=Passthrough  ExternalSaturationOutDataTypeStr=Inherit: Same as second input
  PM Flux1 : Constant  Value=Pm
  Product{9..13} (5 alike) : Product
  Sum : Sum  Inputs=|+-
  Sum1 : Sum  Inputs=++|
  Vd : Outport
  Vq : Outport  Port=2
  wires:
  Ld1/1 -> Product13/2
  Product10/1 -> Sum/2
  Product13/1 -> Add3/1
  PID Controller1/1 -> Sum1/2
  Gain5/1 -> Product11/2
  Sum1/1 -> Vq/1
  Iq_ref/1 -> Add2/1
  omega/1 -> Product11/1
  Lq1/1 -> Product12/2
  Iq/1 -> Product12/1, Add2/2
  PM Flux1/1 -> Add3/2
  Sum/1 -> Vd/1
  Id_ref/1 -> Add1/1
  Product9/1 -> Sum1/1
  Add2/1 -> PID Controller1/1
  Product11/1 -> Product9/1, Product10/2
  Add1/1 -> PID Controller/1
  Number of Poles1/1 -> Gain5/1
  Product12/1 -> Product10/1
  Id/1 -> Add1/2, Product13/1
  PID Controller/1 -> Sum/1
  Add3/1 -> Product9/2

== system Copy_of_vehicle/Motor/FOC/park ==
  I_alpha : Inport
  theta : Inport  Port=2
  I_beta : Inport  Port=3
  Cos : Trigonometry  Operator=cos
  Product{4..7} (4 alike) : Product
  Sin : Trigonometry
  Sum5 : Sum  Inputs=+-
  Sum6 : Sum  Inputs=|++
  Id : Outport
  Iq : Outport  Port=2
  wires:
  Cos/1 -> Product5/2, Product7/2
  Product7/1 -> Sum6/1
  Product6/1 -> Sum6/2
  I_alpha/1 -> Product7/1, Product4/1
  Product5/1 -> Sum5/1
  Sin/1 -> Product4/2, Product6/2
  I_beta/1 -> Product6/1, Product5/1
  Product4/1 -> Sum5/2
  Sum6/1 -> Id/1  "Id"
  Sum5/1 -> Iq/1  "Iq"
  theta/1 -> Cos/1, Sin/1

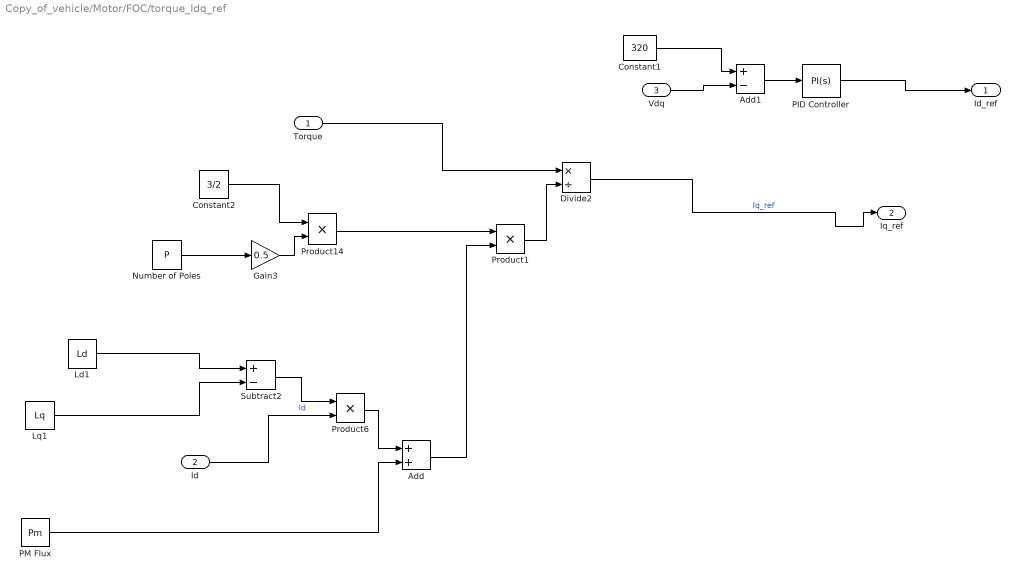
== system Copy_of_vehicle/Motor/FOC/torque_Idq_ref ==
  Torque : Inport
  Id : Inport  Port=2
  Vdq : Inport  Port=3
  Add : Sum
  Add1 : Sum  Inputs=+-
  Constant1 : Constant  Value=320
  Constant2 : Constant  Value=3/2
  Divide2 : Product  Inputs=*/
  Gain3 : Gain  Gain=0.5  OutDataTypeStr=single
  Ld1 : Constant  Value=Ld
  Lq1 : Constant  Value=Lq
  Number of Poles : Constant  Value=P
  PID Controller : pid_lib/PID Controller  Controller=PI  Form=Ideal  TimeDomain=Continuous-time  UseExternalTs=off  SampleTime=Ts  IntegratorMethod=Forward Euler  FilterMethod=Forward Euler  ControllerParametersSource=internal  P=200  I=1  D=0  UseFilter=on  N=100  TunerSelectOption=Transfer Function Based (PID Tuner App)  InitialConditionSource=internal  InitialConditionForIntegrator=0  InitialConditionForFilter=0  DifferentiatorICPrevScaledInput=0  ExternalReset=none  TrackingMode=off  Kt=1  LimitOutput=on  SatLimitsSource=internal  UpperSaturationLimit=0  LowerSaturationLimit=-5  LinearizeAsGain=on  AntiWindupMode=none  Kb=1  POutMin=[]  POutMax=[]  IOutMin=[]  IOutMax=[]  DOutMin=[]  DOutMax=[]  NOutMin=[]  NOutMax=[]  SumOutMin=[]  SumOutMax=[]  SaturationOutMin=[]  SaturationOutMax=[]  PParamMin=[]  PParamMax=[]  IParamMin=[]  IParamMax=[]  DParamMin=[]  DParamMax=[]  NParamMin=[]  NParamMax=[]  KbParamMin=[]  KbParamMax=[]  KtParamMin=[]  KtParamMax=[]  KbOutMin=[]  KbOutMax=[]  KtOutMin=[]  KtOutMax=[]  IntegratorOutMin=[]  IntegratorOutMax=[]  FilterOutMin=[]  FilterOutMax=[]  SumI1OutMin=[]  SumI1OutMax=[]  SumI2OutMin=[]  SumI2OutMax=[]  SumI3OutMin=[]  SumI3OutMax=[]  SumI4OutMin=[]  SumI4OutMax=[]  SumDOutMin=[]  SumDOutMax=[]  DifferentiatorOutMin=[]  DifferentiatorOutMax=[]  FilterDiffOutCoefMin=[]  FilterDiffOutCoefMax=[]  ReciprocalOutMin=[]  ReciprocalOutMax=[]  SumDenOutMin=[]  SumDenOutMax=[]  SumNumOutMin=[]  SumNumOutMax=[]  DivideOutMin=[]  DivideOutMax=[]  UdiffTsProdOutMin=[]  UdiffTsProdOutMax=[]  NTsProdOutMin=[]  NTsProdOutMax=[]  UintegralTsProdOutMin=[]  UintegralTsProdOutMax=[]  UngainTsProdOutMin=[]  UngainTsProdOutMax=[]  IntegratorContinuousStateAttributes=''  IntegratorStateMustResolveToSignalObject=off  IntegratorRTWStateStorageClass=Auto  FilterContinuousStateAttributes=''  FilterStateMustResolveToSignalObject=off  FilterRTWStateStorageClass=Auto  ParallelPVariant=Passthrough  IdealPVariant=InternalParameters  IVariant=InternalParameters  DVariant=Disabled  IntegratorVariant=Continuous  SatVariant=Enabled  AWVariant=Passthrough  PCopyVariant=Disabled  TRVariant=Disabled  FdbkBlocksVariant=Forward  IdealPFdbkVariant=Disabled  SatFdbkVariant=Disabled  DerivativeFilterVariant=Disabled  NVariant=Disabled  NCopyVariant=Disabled_SignalSpec  FilterICVariant=Disabled  IntegratorICVariant=InternalICs  ExternalResetVariant=Disabled  TRSumVariant=Passthrough  SumFdbkVariant=Disabled  SumVariant=Sum_PI  TsampFilterVariant=InternalTs  TsampNgainVariant=Passthrough  TsampIntegralVariant=Passthrough  ExternalSaturationOutDataTypeStr=Inherit: Same as second input
  PM Flux : Constant  Value=Pm
  Product1 : Product
  Product14 : Product
  Product6 : Product
  Subtract2 : Sum  Inputs=+-
  Id_ref : Outport
  Iq_ref : Outport  Port=2
  wires:
  Product1/1 -> Divide2/2
  Gain3/1 -> Product14/2
  Lq1/1 -> Subtract2/2
  Number of Poles/1 -> Gain3/1
  Subtract2/1 -> Product6/1
  Ld1/1 -> Subtract2/1
  Add/1 -> Product1/2
  Product6/1 -> Add/1
  Constant2/1 -> Product14/1
  Product14/1 -> Product1/1
  Divide2/1 -> Iq_ref/1  "Iq_ref"
  PM Flux/1 -> Add/2
  Id/1 -> Product6/2  "Id"
  Constant1/1 -> Add1/1
  Torque/1 -> Divide2/1
  Vdq/1 -> Add1/2
  Add1/1 -> PID Controller/1
  PID Controller/1 -> Id_ref/1

== system Copy_of_vehicle/Motor/PMSM/Inverse - Park1 ==
  Id : Inport
  Iq : Inport  Port=2
  theta : Inport  Port=3
  Cos : Trigonometry  Operator=cos
  Product{,1..3} (4 alike) : Product
  Sin : Trigonometry
  Sum3 : Sum  Inputs=|++
  Sum4 : Sum  Inputs=+-
  I-alpha : Outport
  I-beta : Outport  Port=2
  wires:
  Iq/1 -> Product2/1, Product1/1
  Cos/1 -> Product1/2, Product3/2
  Sin/1 -> Product2/2, Product/2
  Product/1 -> Sum3/2
  Product3/1 -> Sum4/1
  Sum3/1 -> I-beta/1
  Product1/1 -> Sum3/1
  Product2/1 -> Sum4/2
  Id/1 -> Product/1, Product3/1
  Sum4/1 -> I-alpha/1
  theta/1 -> Cos/1, Sin/1

== system Copy_of_vehicle/Motor/PMSM/Inverse Clarke1 ==
  Ialpha : Inport
  Ibeta : Inport  Port=2
  Constant : Constant  Value=0.5  OutDataTypeStr=single
  Constant18 : Constant  Value=3/4  OutDataTypeStr=single
  Product8 : Product
  Product9 : Product
  Sqrt : Sqrt  SaturateOnIntegerOverflow=on
  Sum : Sum  Inputs=-+
  Sum1 : Sum  Inputs=--
  Sum7 : Sum  Inputs=|++
  Ia : Outport
  Ib : Outport  Port=2
  Ic : Outport  Port=3
  wires:
  Product9/1 -> Sum1/2, Sum/2
  Product8/1 -> Sum7/1, Sum1/1, Sum7/2, Sum/1
  Constant18/1 -> Sqrt/1
  Sum/1 -> Ib/1
  Ibeta/1 -> Product9/1
  Sum7/1 -> Ia/1
  Constant/1 -> Product8/2
  Sqrt/1 -> Product9/2
  Sum1/1 -> Ic/1
  Ialpha/1 -> Product8/1

== system Copy_of_vehicle/Motor/PMSM/Subsystem1 ==
  omega : Inport
  Constant8 : Constant  Value=2*pi
  Gain4 : Gain  Gain=0.5
  Integrator2 : Integrator
  Math Function : Math  Operator=mod  SaturateOnIntegerOverflow=on
  Number of Poles1 : Constant  Value=P
  Product15 : Product
  Unit Delay : UnitDelay  SampleTime=Ts  HasFrameUpgradeWarning=on
  theta : Outport
  wires:
  Constant8/1 -> Math Function/2
  Number of Poles1/1 -> Gain4/1
  Math Function/1 -> theta/1
  Unit Delay/1 -> Integrator2/1
  Integrator2/1 -> Product15/1
  Gain4/1 -> Product15/2
  Product15/1 -> Math Function/1
  omega/1 -> Unit Delay/1

== system Copy_of_vehicle/Motor/PMSM/Subsystem2 ==
  Iq : Inport
  Id : Inport  Port=2
  Add : Sum
  Constant : Constant  Value=3/2
  Gain : Gain  Gain=0.5
  Number of Poles1 : Constant  Value=P
  Number of Poles2 : Constant  Value=Ld
  Number of Poles3 : Constant  Value=Lq
  Number of Poles4 : Constant  Value=Pm
  Product5 : Product  Inputs=4
  Product6 : Product
  Subtract2 : Sum  Inputs=+-
  Torque : Outport
  wires:
  Add/1 -> Product5/4
  Gain/1 -> Product5/2
  Product6/1 -> Add/1
  Number of Poles4/1 -> Add/2
  Number of Poles2/1 -> Subtract2/1
  Number of Poles1/1 -> Gain/1
  Number of Poles3/1 -> Subtract2/2
  Constant/1 -> Product5/1
  Id/1 -> Product6/2
  Subtract2/1 -> Product6/1
  Iq/1 -> Product5/3
  Product5/1 -> Torque/1

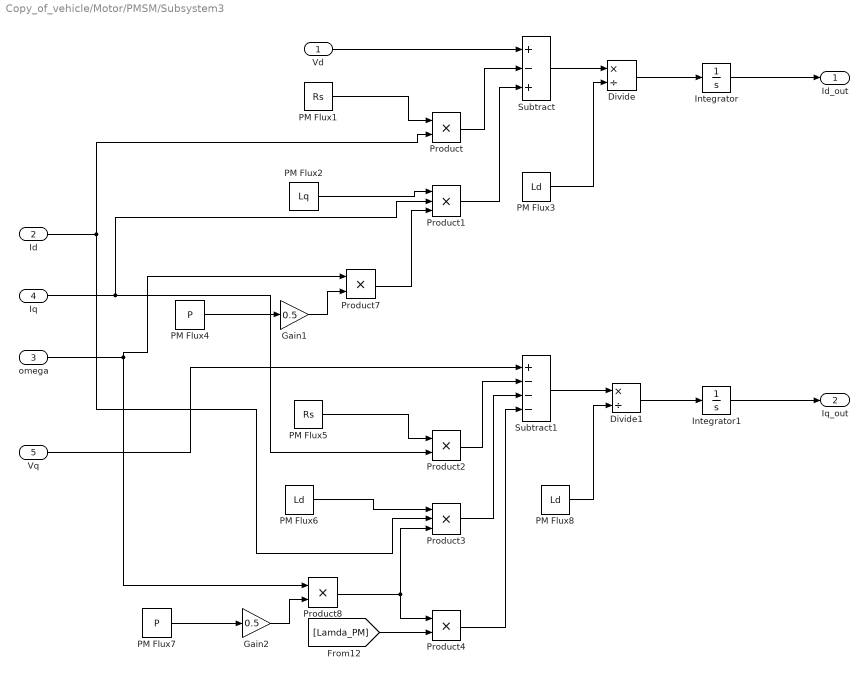
== system Copy_of_vehicle/Motor/PMSM/Subsystem3 ==
  Vd : Inport
  Id : Inport  Port=2
  omega : Inport  Port=3
  Iq : Inport  Port=4
  Vq : Inport  Port=5
  Divide : Product  Inputs=*/
  Divide1 : Product  Inputs=*/
  Gain1 : Gain  Gain=0.5
  Gain2 : Gain  Gain=0.5
  Integrator : Integrator
  Integrator1 : Integrator
  PM Flux1 : Constant  Value=Rs
  PM Flux2 : Constant  Value=Lq
  PM Flux3 : Constant  Value=Ld
  PM Flux4 : Constant  Value=P
  PM Flux5 : Constant  Value=Rs
  PM Flux6 : Constant  Value=Ld
  PM Flux7 : Constant  Value=P
  PM Flux8 : Constant  Value=Ld
  Product{,2,4,7..8} (5 alike) : Product
  Product1 : Product  Inputs=3
  Product3 : Product  Inputs=3
  Subtract : Sum  Inputs=+-+
  Subtract1 : Sum  Inputs=+---
  Id_out : Outport
  Iq_out : Outport  Port=2
  wires:
  PM Flux6/1 -> Product3/1
  PM Flux5/1 -> Product2/1
  Gain1/1 -> Product7/2
  Id/1 -> Product/2, Product3/2
  Product4/1 -> Subtract1/4
  Iq/1 -> Product2/2, Product1/2
  PM Flux3/1 -> Divide/2
  PM Flux1/1 -> Product/1
  omega/1 -> Product7/1, Product8/1
  PM Flux4/1 -> Gain1/1
  Subtract1/1 -> Divide1/1
  PM Flux2/1 -> Product1/1
  Integrator/1 -> Id_out/1
  Product8/1 -> Product3/3, Product4/1
  Divide/1 -> Integrator/1
  Product7/1 -> Product1/3
  Subtract/1 -> Divide/1
  Product/1 -> Subtract/2
  Gain2/1 -> Product8/2
  Product3/1 -> Subtract1/3
  Integrator1/1 -> Iq_out/1
  Divide1/1 -> Integrator1/1
  [Lamda_PM] -> Product4/2
  PM Flux8/1 -> Divide1/2
  Product1/1 -> Subtract/3
  Product2/1 -> Subtract1/2
  PM Flux7/1 -> Gain2/1
  Vq/1 -> Subtract1/1
  Vd/1 -> Subtract/1

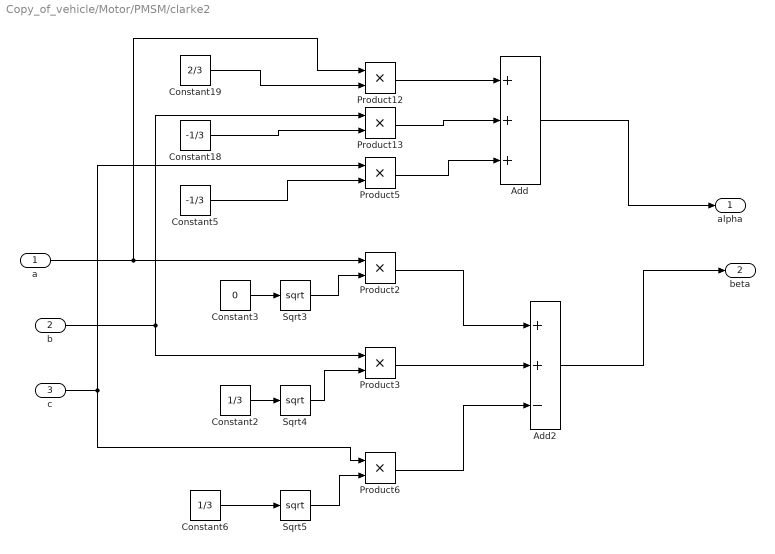
== system Copy_of_vehicle/Motor/PMSM/clarke2 ==
  a : Inport
  b : Inport  Port=2
  c : Inport  Port=3
  Add : Sum  Inputs=+++
  Add2 : Sum  Inputs=++-
  Constant18 : Constant  Value=-1/3  OutDataTypeStr=single
  Constant19 : Constant  Value=2/3  OutDataTypeStr=single
  Constant2 : Constant  Value=1/3  OutDataTypeStr=single
  Constant3 : Constant  Value=0  OutDataTypeStr=single
  Constant5 : Constant  Value=-1/3  OutDataTypeStr=single
  Constant6 : Constant  Value=1/3  OutDataTypeStr=single
  Product{2..3,5..6,12..13} (6 alike) : Product
  Sqrt3 : Sqrt  SaturateOnIntegerOverflow=on
  Sqrt4 : Sqrt  SaturateOnIntegerOverflow=on
  Sqrt5 : Sqrt  SaturateOnIntegerOverflow=on
  alpha : Outport
  beta : Outport  Port=2
  wires:
  Constant19/1 -> Product12/2
  Constant18/1 -> Product13/2
  Constant3/1 -> Sqrt3/1
  Sqrt4/1 -> Product3/2
  Constant2/1 -> Sqrt4/1
  Sqrt3/1 -> Product2/2
  a/1 -> Product12/1, Product2/1
  b/1 -> Product3/1, Product13/1
  Constant5/1 -> Product5/2
  c/1 -> Product6/1, Product5/1
  Constant6/1 -> Sqrt5/1
  Sqrt5/1 -> Product6/2
  Product12/1 -> Add/1
  Product13/1 -> Add/2
  Product2/1 -> Add2/1
  Product3/1 -> Add2/2
  Product6/1 -> Add2/3
  Add/1 -> alpha/1
  Add2/1 -> beta/1
  Product5/1 -> Add/3

== system Copy_of_vehicle/Motor/PMSM/park ==
  V-alpha : Inport
  V-beta : Inport  Port=2
  theta : Inport  Port=3
  Cos : Trigonometry  Operator=cos
  Product{4..7} (4 alike) : Product
  Sin : Trigonometry
  Sum5 : Sum  Inputs=+-
  Sum6 : Sum  Inputs=|++
  Vd : Outport
  Vq : Outport  Port=2
  wires:
  Cos/1 -> Product5/2, Product7/2
  Product7/1 -> Sum6/1
  Product6/1 -> Sum6/2
  V-alpha/1 -> Product4/1, Product7/1
  Product5/1 -> Sum5/1
  Sin/1 -> Product6/2, Product4/2
  V-beta/1 -> Product5/1, Product6/1
  Product4/1 -> Sum5/2
  Sum6/1 -> Vd/1
  Sum5/1 -> Vq/1
  theta/1 -> Cos/1, Sin/1

== system Copy_of_vehicle/Vehicle Control Unit/Cruise Control1/Capture speed ==
  Vveh : Inport
  Trigger : TriggerPort  VariantControl=Variant
  Vref : Outport  VectorParamsAs1DForOutWhenUnconnected=off
  wires:
  Vveh/1 -> Vref/1

== system Copy_of_vehicle/Vehicle Control Unit/Cruise Control1/Inputs1 ==
  Demux : Demux  Tag=STV Demux  Outputs=2
      settings: DisplayOption=none
  FromWs : FromWorkspace  Tag=STV FromWs  VariableName=tuvar  SampleTime=0.01
      SigBuilderData=|
      | common.afterFinalStr = 'Extrapolate'
      | common.sampleTime = '0.01'
      | dataSet.timeRange = [0 200]
      | dataSet.name = 'Test 1'
      | sbobj.Name = 'Signal Builder'
      | sbobj.Groups.Name = 'Test 1'
      | sbobj.Groups.Signals(1).Name = 'Cruise Ena.'
      | sbobj.Groups.Signals(1).XData = [0 8 24.5 200]
      | sbobj.Groups.Signals(1).YData = [0 0 0 0]
      | sbobj.Groups.Signals(2).Name = 'Cruise Dis.'
      | sbobj.Groups.Signals(2).XData = [0 200]
      | sbobj.Groups.Signals(2).YData = [0 0]
      | sbobj.Groups.TimeRange = [0 200]
  Cruise Ena. : Outport  Tag=STV Outport  VectorParamsAs1DForOutWhenUnconnected=off
  Cruise Dis. : Outport  Tag=STV Outport  Port=2  VectorParamsAs1DForOutWhenUnconnected=off
  wires:
  FromWs/1 -> Demux/1
  Demux/1 -> Cruise Ena./1
  Demux/2 -> Cruise Dis./1

== system Copy_of_vehicle/Vehicle Control Unit/Cruise Control1/Subsystem ==
  Acc_pedal : Inport
  velocity : Inport  Port=2
  1-D Lookup Table1 : Lookup_n-D  NumberOfTableDimensions=1  BreakpointsForDimension1=[0 , 27.78,50]  Table=T_lookup  InternalRulePriority=Speed  RndMeth=Simplest  InputSameDT=on
  Product1 : Product
  Torque_cmd : Outport
  wires:
  Acc_pedal/1 -> Product1/1
  1-D Lookup Table1/1 -> Product1/2
  Product1/1 -> Torque_cmd/1
  velocity/1 -> 1-D Lookup Table1/1

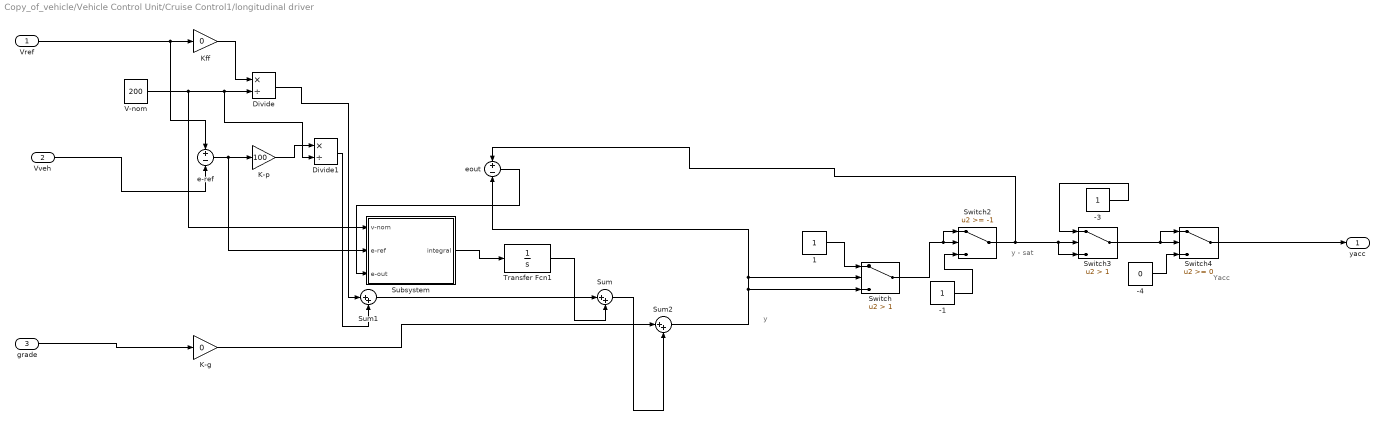
== system Copy_of_vehicle/Vehicle Control Unit/Cruise Control1/longitudinal driver ==
  note: Yacc
  note: y - sat
  note: y
  Vref : Inport
  Vveh : Inport  Port=2
  grade : Inport  Port=3
  -1 : Constant
  -3 : Constant
  -4 : Constant  Value=0
  1 : Constant
  Divide : Product  Inputs=*/
  Divide1 : Product  Inputs=*/
  K-g : Gain  Gain=0
  K-p : Gain  Gain=100
  Kff : Gain  Gain=0
  Subsystem : Subsystem
  Sum : Sum  Inputs=|++
  Sum1 : Sum  Inputs=|++
  Sum2 : Sum  Inputs=|++
  Switch : Switch  Criteria=u2 > Threshold  Threshold=1
  Switch2 : Switch  Threshold=-1
  Switch3 : Switch  Criteria=u2 > Threshold  Threshold=1
  Switch4 : Switch
  Transfer Fcn1 : TransferFcn  Denominator=[1 0]
  V-nom : Constant  Value=200
  e-ref : Sum  Inputs=+-
  eout : Sum  Inputs=+-
  yacc : Outport
  wires:
  1/1 -> Switch/1
  Switch4/1 -> yacc/1
  V-nom/1 -> Divide1/2, Divide/2, Subsystem/1(v-nom)
  Switch2/1 -> Switch3/3, Switch3/2, eout/1
  e-ref/1 -> Subsystem/2(e-ref), K-p/1
  Sum/1 -> Sum2/2
  -3/1 -> Switch3/1
  -4/1 -> Switch4/3
  Switch/1 -> Switch2/1, Switch2/2
  Divide/1 -> Sum1/1
  -1/1 -> Switch2/3
  Sum2/1 -> Switch/3, eout/2, Switch/2
  Vref/1 -> e-ref/1, Kff/1
  Subsystem/1(integral) -> Transfer Fcn1/1
  K-p/1 -> Divide1/1
  Sum1/1 -> Sum/1
  Switch3/1 -> Switch4/1, Switch4/2
  Transfer Fcn1/1 -> Sum/2
  Kff/1 -> Divide/1
  eout/1 -> Subsystem/3(e-out)
  Vveh/1 -> e-ref/2
  K-g/1 -> Sum2/1
  Divide1/1 -> Sum1/2
  grade/1 -> K-g/1

== system Copy_of_vehicle/Vehicle Control Unit/Cruise Control1/longitudinal driver/Subsystem ==
  v-nom : Inport
  e-ref : Inport  Port=2
  e-out : Inport  Port=3
  Divide2 : Product  Inputs=*/
  K-aw : Gain  Gain=0
  Ki : Gain
  Sum2 : Sum  Inputs=|++
  integral : Outport
  wires:
  Divide2/1 -> Sum2/1
  v-nom/1 -> Divide2/2
  e-ref/1 -> Ki/1
  K-aw/1 -> Sum2/2
  Ki/1 -> Divide2/1
  e-out/1 -> K-aw/1
  Sum2/1 -> integral/1
